simulink model "OFDM"  (R2019a)
settings: Solver=FixedStepDiscrete  StartTime=0.0  StopTime=inf  RelTol=1e-3
PreLoadFcn:
  | %global Ts
  | %global nbSymboles
  | %global ratioPiloSymb
  | %global puissanceDeDeux
  | %global nbPilotes
  | %global nbZeros
  | %global nbDeBits
  | 
  | clear all;
  | 
  | Ts = 6e-6;
  | nbDeBits = 180
  | nbSymboles = nbDeBits/2
  | ratioPiloSymb = 3
  | puissanceDeDeux = 128
  | 
  | nbPilotes = nbSymboles/ratioPiloSymb;
  | nbZeros = puissanceDeDeux - nbSymboles - nbPilotes
InitFcn:
  | %global Ts
  | %global nbSymboles
  | %global ratioPiloSymb
  | %global puissanceDeDeux
  | %global nbPilotes
  | %global nbZeros
  | %global nbDeBits
  | 
  | clear all;
  | 
  | Ts = 6e-6;
  | nbDeBits = 400
  | nbSymboles = nbDeBits/2
  | ratioPiloSymb = 20
  | puissanceDeDeux = 256
  | 
  | nbPilotes = nbSymboles/ratioPiloSymb;
  | nbZeros = puissanceDeDeux - nbSymboles - nbPilotes
model workspace (MAT data in the model file):
  Var = Simulink.Parameter
  Var.Value = 180
  Var.DataType = 'auto'
  Var.Dimensions = [1 1]
undefined symbols (not defined in the file): doppler
libraries: dspxfrm3 x2, commdigbbndpm3 x2, commrandsrc3 x1, commsink2 x1, commutil2 x1, commchan3 x1
settings Model: OrderedModelArguments=off  Creator=coco  LastModifiedBy=julien
settings SolverCC: AutoInsertRateTranBlk=on
settings DataIOCC: LimitDataPoints=on  SaveOutput=off  SignalLogging=off  SaveTime=off
settings OptimizationCC: LifeSpan=inf
settings DebuggingCC: AlgebraicLoopMsg=error  SingleTaskRateTransMsg=error  AllowSymbolicDim=off  SFUnexpectedBacktrackingDiag=warning  SFNoUnconditionalDefaultTransitionDiag=warning  SFExecutionAtInitializationDiag=none  ArithmeticOperatorsInVariantConditions=warning
settings SFSimCC: SimUseLocalCustomCode=off
settings RTWCC: RTWUseLocalCustomCode=off
settings CodeAppCC: StateflowObjectComments=on
settings GRTTargetCC: TargetLangStandard=C89/C90 (ANSI)  GeneratePreprocessorConditionals=Disable all

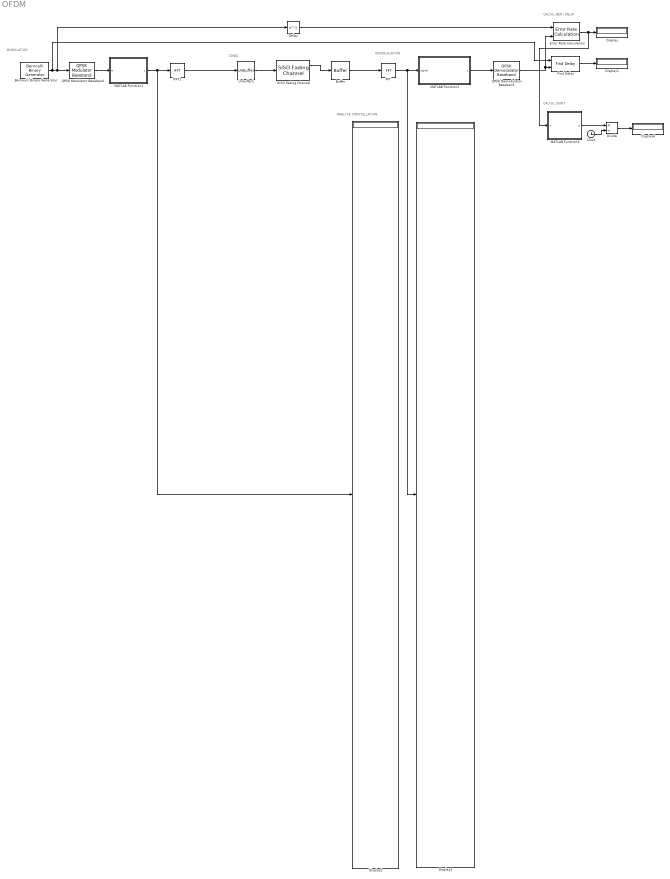
== system OFDM ==
  note: ANALYSE CONSTELLATION
  note: CALCUL DEBIT
  note: CALCUL BER / DELAI
  note: MODULATION
  note: CANAL
  note: DEMODULATION
  Bernoulli Binary Generator : commrandsrc3/Bernoulli Binary Generator  ProbabilityOfZero=0.5  SeedSource=Auto  Seed=0  SampleTime=Ts/nbDeBits  SamplesPerFrame=nbDeBits  OutputDataType=double  SimulateUsing=Interpreted execution
      settings: SourceProductName=Communications Toolbox
  Buffer : Buffer  N=puissanceDeDeux  OutputFrames=off
  Clock : Clock
  Delay : Delay  DelayLength=1  InitialCondition=0
  Display{,1..4} (5 alike) : Display
  Divide : Product  Inputs=*/  SaturateOnIntegerOverflow=on  RndMeth=Zero
  Error Rate Calculation : commsink2/Error Rate Calculation  N=0  st_delay=0  cp_mode=Entire frame  subframe=[]  PMode=Port  WsName=ErrorVec  RsMode2=off  stop=off  numErr=100  maxBits=1e6
      settings: SourceProductName=Communications Toolbox
  FFT : dspxfrm3/FFT  FFTImplementation=Auto  CompMethod=Table lookup  TableOpt=NEW  TableOptActive=Speed  BitRevOrder=off  Normalize=off  InheritFFTLength=on  FFTLength=64  WrapInput=on  roundingMode=Floor  overflowMode=off  firstCoeffDataTypeStr=Inherit: Same word length as input  firstCoeffLastDataTypeStr=Inherit: Same word length as input  outputMin=[]  outputMax=[]
  Find Delay : commutil2/Find Delay  corrLength=180  chgSigOP=off  stopUpdate=off  numConstDelay=3
      settings: SourceProductName=Communications Toolbox  SourceProductBaseCode=CM
  IFFT1 : dspxfrm3/IFFT  FFTImplementation=Auto  CompMethod=Table lookup  TableOpt=NEW  TableOptActive=Speed  BitRevOrder=off  cs_in=off  Normalize=on  InheritFFTLength=on  FFTLength=64  WrapInput=on  mode=Complex  outSamplingMode=Sample based  roundingMode=Floor  overflowMode=off  firstCoeffDataTypeStr=Inherit: Same word length as input  firstCoeffLastDataTypeStr=Inherit: Same word length as input  outputMin=[]  outputMax=[]
      settings: SourceProductName=DSP System Toolbox
  MATLAB Function1 : MATLAB Function  TreatAsAtomicUnit=on
  MATLAB Function2 : MATLAB Function  TreatAsAtomicUnit=on
  MATLAB Function3 : MATLAB Function  TreatAsAtomicUnit=on
  QPSK Demodulator Baseband : commdigbbndpm3/QPSK Demodulator Baseband  OutType=Bit  DecType=Hard decision  VarSource=Dialog  Variance=1  Dec=Gray  Ph=pi/4  outDtype1=Inherit via internal rule  outDtype2=Inherit via internal rule  derotateFactorWordLen=16  derotateFactorDataTypeStr=Inherit: Same word length as input  derotateFactorLastDataTypeStr=Inherit: Same word length as input
      settings: SourceProductName=Communications Toolbox
  QPSK Modulator Baseband : commdigbbndpm3/QPSK Modulator Baseband  InType=Bit  Enc=Gray  Ph=pi/4  outDtype=double  outWordLen=16  outUDDataType=sfix(16)  outFracLenMode=Best precision  outFracLen=15  outDataTypeStr=double  outLastDataTypeStr=double
      settings: SourceProductName=Communications Toolbox
  SISO Fading Channel : commchan3/SISO Fading Channel  InheritSampleRate=on  SampleRate=1  PathDelays=[0 (6e-6/128)*2 (6e-6/128)*4]  AveragePathGains=[0 -3 -6]  NormalizePathGains=on  FadingDistribution=Rayleigh  KFactor=3  DirectPathDopplerShift=0  DirectPathInitialPhase=0  MaximumDopplerShift=10  DopplerSpectrum=doppler('Jakes')  ChannelInterpolationMethod=Polyphase  RandomStream=mt19937ar with seed  RandomNumGenerator=mt19937ar  Seed=73  PathGainsOutputPort=on  ChannelFilterDelayOutputPort=off  SimulateUsing=Interpreted execution  Visualization=Off  PathsForDopplerDisplay=1  SamplesToDisplay=25%
      settings: SourceProductName=Communications Toolbox
  Unbuffer1 : Unbuffer  ic=puissanceDeDeux
  wires:
  Unbuffer1/1 -> SISO Fading Channel/1
  SISO Fading Channel/1 -> Buffer/1
  Buffer/1 -> FFT/1
  QPSK Demodulator Baseband/1 -> Find Delay/2, Error Rate Calculation/2
  IFFT1/1 -> Unbuffer1/1
  Bernoulli Binary Generator/1 -> Find Delay/1, Delay/1, QPSK Modulator Baseband/1
  Delay/1 -> Error Rate Calculation/1
  Find Delay/1 -> Display1/1
  QPSK Modulator Baseband/1 -> MATLAB Function1/1(a)
  FFT/1 -> Display3/1, MATLAB Function2/1(signal)
  MATLAB Function1/1(z) -> Display2/1, IFFT1/1
  MATLAB Function2/1(z) -> QPSK Demodulator Baseband/1
  Divide/1 -> Display4/1
  Clock/1 -> Divide/2
  Error Rate Calculation/1 -> MATLAB Function3/1(x), Display/1
  MATLAB Function3/1(y) -> Divide/1

== matlab function OFDM/MATLAB Function1 ==
  data: z output; a input; puissanceDeDeux parameter; nbZeros parameter; nbSymboles parameter; ratioPiloSymb parameter
function z = AjoutPilotesZeros(a, puissanceDeDeux, nbZeros, nbSymboles, ratioPiloSymb)

z = complex(zeros(puissanceDeDeux,1));

k = 1;

for p = 1:nbSymboles
    if p == nbSymboles/2 + 1
        z(k : k+nbZeros) = 0;
        k = k + nbZeros;
    end
    if mod(p,ratioPiloSymb) == 1
        z(k) = 1;
        k = k + 1;
    end
    z(k) = a(p);
    k = k + 1;
end

== matlab function OFDM/MATLAB Function3 ==
  data: x input; y output
function y = CalculDebit(x)
y = x(3) - x(2);

== matlab function OFDM/MATLAB Function2 ==
  data: signal input; z output; puissanceDeDeux parameter; nbZeros parameter; nbSymboles parameter; ratioPiloSymb parameter
function z = SuppPilotesZerosEgalisation(signal, puissanceDeDeux, nbZeros, nbSymboles, ratioPiloSymb)

z = complex(zeros(nbSymboles,1));

k = 1;

gain = 0;

shift = 0; % Détermine dans si les 0 ont été franchis ou non.

for p = 1:nbSymboles
    if k == (puissanceDeDeux)/2 - round(nbZeros/2) +1
        k = k + nbZeros;
        shift = 1;
    end
    if (mod(k-nbZeros,ratioPiloSymb + 1) == 1) && (shift == 1)
        gain = signal(k);
        k = k + 1;
    end
    if (mod(k,ratioPiloSymb + 1) == 1) && (shift == 0)
        gain = signal(k);
        k = k + 1;
    end
    z(p) = signal(k)/gain;
    k = k + 1;
end
